simulink model "Demo_TA_cs"  (R2014b)
settings: Solver=FixedStepDiscrete  StartTime=0.0  StopTime=5  FixedStep=1/60  RelTol=1e-3
PreLoadFcn:
  | mbxruntime.callbacks.PreLoadFcn(bdroot);
  | check_NUTS_defined
  | 
  | assignin('base',['model_closed_' bdroot],false);
PostLoadFcn:
  | mbxruntime.callbacks.PostLoadFcn(bdroot);
InitFcn:
  | mbxruntime.callbacks.InitFcn(bdroot);
StartFcn:
  | mbxruntime.callbacks.StartFcn(bdroot);
  | 
  | open_system([bdroot '/Mazda_RX8_1/Scope']);
StopFcn:
  | mbxruntime.callbacks.StopFcn(bdroot);;
  | 
model workspace: external: MAT-File .\Demo_TA_cs_hws.mat (data not in the file)
undefined symbols (not defined in the file or in its folder): DriftAzimuthGaussianSigma, DriftAzimuthGaussianSigmaDefined, NoiseAzimuthIllumination, NoiseAzimuthIlluminationDefined, NoiseAzimuthReflection, NoiseAzimuthReflectionDefined, NoiseRange, NoiseRangeDefined, NoiseRangeType, NoiseRangeTypeDefined
undefined symbols (not defined in the file): Demo_TA_cs_Box_1_Dynamics_Empty_STATE_Box_1_Pitch0, Demo_TA_cs_Box_1_Dynamics_Empty_STATE_Box_1_Roll0, Demo_TA_cs_Box_1_Dynamics_Empty_STATE_Box_1_x0, Demo_TA_cs_Box_1_Dynamics_Empty_STATE_Box_1_y0, Demo_TA_cs_Box_1_Dynamics_Empty_STATE_Box_1_Yaw0, Demo_TA_cs_Box_1_Dynamics_Empty_STATE_Box_1_z0, Demo_TA_cs_Box_2_Dynamics_Empty_STATE_Box_2_Pitch0, Demo_TA_cs_Box_2_Dynamics_Empty_STATE_Box_2_Roll0, Demo_TA_cs_Box_2_Dynamics_Empty_STATE_Box_2_x0, Demo_TA_cs_Box_2_Dynamics_Empty_STATE_Box_2_y0, Demo_TA_cs_Box_2_Dynamics_Empty_STATE_Box_2_Yaw0, Demo_TA_cs_Box_2_Dynamics_Empty_STATE_Box_2_z0, Demo_TA_cs_Box_3_Dynamics_Empty_STATE_Box_3_Pitch0, Demo_TA_cs_Box_3_Dynamics_Empty_STATE_Box_3_Roll0, Demo_TA_cs_Box_3_Dynamics_Empty_STATE_Box_3_x0, Demo_TA_cs_Box_3_Dynamics_Empty_STATE_Box_3_y0, Demo_TA_cs_Box_3_Dynamics_Empty_STATE_Box_3_Yaw0, Demo_TA_cs_Box_3_Dynamics_Empty_STATE_Box_3_z0, Demo_TA_cs_Mazda_RX8_1_Dynamics_Empty_STATE_Mazda_RX8_1_Pitch0, Demo_TA_cs_Mazda_RX8_1_Dynamics_Empty_STATE_Mazda_RX8_1_Roll0, Demo_TA_cs_Mazda_RX8_1_Dynamics_Empty_STATE_Mazda_RX8_1_x0, Demo_TA_cs_Mazda_RX8_1_Dynamics_Empty_STATE_Mazda_RX8_1_y0, Demo_TA_cs_Mazda_RX8_1_Dynamics_Empty_STATE_Mazda_RX8_1_Yaw0, Demo_TA_cs_Mazda_RX8_1_Dynamics_Empty_STATE_Mazda_RX8_1_z0
libraries: PreScanSimulinkLibrary x8, PreScanUsefulBlocks x1
(part 1 of 2)
CloseFcn:
  | mbxruntime.callbacks.CloseFcn(bdroot);
  | evalin('base',['clear model_closed_' bdroot]);
settings Model: Creator=PRESCAN  LastModifiedBy=jenkins
settings DataIOCC: SignalLoggingSaveFormat=ModelDataLogs
settings OptimizationCC: InlineParams=on  ExpressionDepthLimit=2147483647  InitFltsAndDblsToZero=on
settings DebuggingCC: SaveWithParameterizedLinksMsg=none  UnderspecifiedInitializationDetection=Classic  MergeDetectMultiDrivingBlocksExec=none  SignalResolutionControl=TryResolveAllWithWarning  SolverPrmCheckMsg=none  MultiTaskDSMMsg=warning  MultiTaskCondExecSysMsg=none  FcnCallInpInsideContextMsg=UseLocalSettings  StateNameClashWarn=warning
settings ModelReferenceCC: UpdateModelReferenceTargets=IfOutOfDate
settings SFSimCC: SimParseCustomCode=off
settings SFSimCC: SimCustomHeaderCode=|
  | #include "prescan.h"
  | #include "prescan_platform.h"
settings RTWCC: IncludeERTFirstTime=on
settings GRTTargetCC: TargetFcnLib=ansi_tfl_tmw.mat  CombineOutputUpdateFcns=off  GRTInterface=on

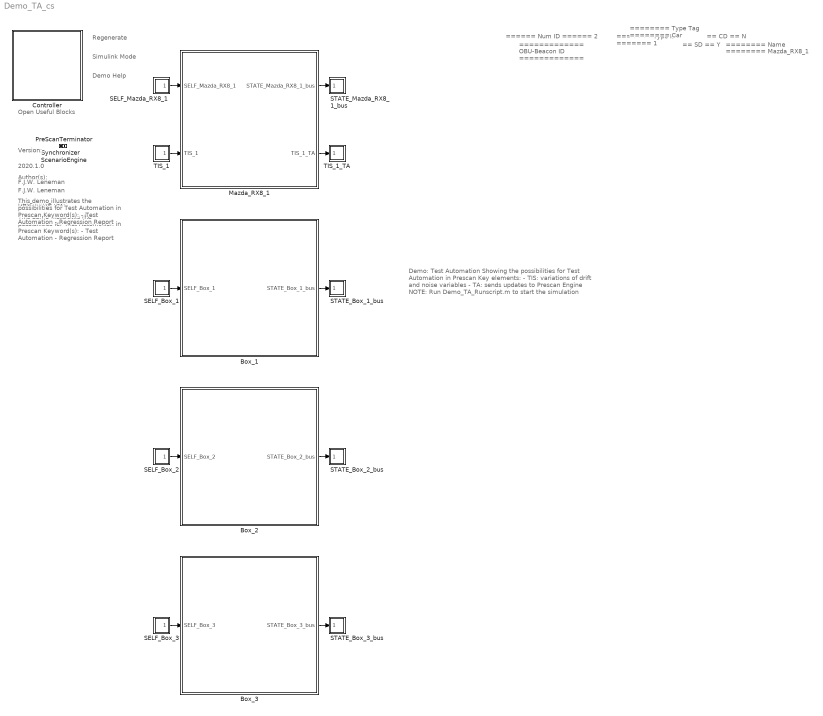
== system Demo_TA_cs ==
  note: Regenerate
  note: Simulink Mode
  note: Open Useful Blocks
  note: 2020.1.0
  note: Version:
  note: Author(s):
  note: F.J.W. Leneman
  note: Descriptive text:
  note: This demo illustrates the
      | possibilities for Test Automation
      | in Prescan
      |
      |
      |
      | Keyword(s):
      |
      | - Test Automation
      |
      | - Regression Report
  note: Demo Help
  note: Demo: Test Automation
      | Showing the possibilities for Test Automation in Prescan
      |
      | Key elements:
      | - TIS: variations of drift and noise variables
      | - TA: sends updates to Prescan Engine
      |
      | NOTE:
      | Run Demo_TA_Runscript.m to start the simulation
  note: This demo illustrates the
      | possibilities for Test Automation
      | in Prescan
      |
      |
      |
      | Keyword(s):
      |
      | - Test Automation
      |
      | - Regression Report
  note: F.J.W. Leneman
  note: ======
      | Num ID
      | ======
      | 2
  note: =============
      | OBU-Beacon ID
      | =============
  note: =======
      | Type ID
      | =======
      | 1
  note: ========
      | Type Tag
      | ========
      | Car
  note: ==
      | SD
      | ==
      | Y
  note: ==
      | CD
      | ==
      | N
  note: ========
      | Name
      | ========
      | Mazda_RX8_1
  Box_1 : Subsystem  Tag=WorldObjectSubSystem  InitFcn=UniqueId = '8';
      mask init:
      | imagePath=which('Box.jpg');
      mask Display: image(imread(imagePath));color('white');text(0, 0, ' ID=3\n')
  Box_2 : Subsystem  Tag=WorldObjectSubSystem  InitFcn=UniqueId = '9';
      mask init:
      | imagePath=which('Box.jpg');
      mask Display: image(imread(imagePath));color('white');text(0, 0, ' ID=4\n')
  Box_3 : Subsystem  Tag=WorldObjectSubSystem  InitFcn=UniqueId = '10';
      mask init:
      | imagePath=which('Box.jpg');
      mask Display: image(imread(imagePath));color('white');text(0, 0, ' ID=5\n')
  Controller : Subsystem  Description=8A3CD2955739A82C886C20AE3E253D78460D53180EE2C1B14CC08DF75A70BE77  Priority=-1  LoadFcn=load PreScanControllerData  mask(PreScan Simulation Controller){prescanversion='2020.1.0', ModelReferencing=off, TimeStep=1/60, ControlMode=0, PreScanExecutionMode=on, ControllerCount=0, ControllerIndex=0, ControllerOptions=''}
      mask prompts: prescanversion "PreScan Version"; ModelReferencing "Use Model Referencing"; TimeStep "Upload Period [s]"; ControlMode "Control Mode"; PreScanExecutionMode "Execution Mode"; ControllerCount "Controller Count"; ControllerIndex "Controller Index"; ControllerOptions "Controller Options"
      mask help:
      | Please do not remove this block from the compilation sheet,
      | as it connects the model to the PreScan environment.
      mask init:
      | model = bdroot(gcb);
      | ExperimentFile = mbxruntime.findExperimentFile(model,true); %relative path
      | 
      | [d1, d2, d3, prescandata] = prescan_Settings();
      | ModelDepo = fullfile(prescandata,'ModelDepo'); 
      | 
      | RTmode = mbxruntime.getRTMode(model);
      | 
      | SimulationMode = get_param(bdroot,'SimulationMode');
      | if strcmp(SimulationMode, 'rapid-accelerator')
      |     SimulationMode = 'external';
      | end
      | TargetName = get_param(bdroot,'SystemTargetFile');
      settings: ModelCloseFcn=assignin('base',['model_closed_' bdroot],true);
      mask Help: eval('openHelp(812)')
      mask Display: image(imread('prescanlogo.ico'))
  Mazda_RX8_1 : Subsystem  Tag=WorldObjectSubSystem  InitFcn=UniqueId = '6';
      mask init:
      | modelPath = GenericModelHelper.getGenericModelFilePath('ModelDepo','Vehicles\Mazda_RX8\Mazda_RX8.pgmb','1e55a2e40efa576b7f4fb93bae35d605');imagePath = GenericModelHelper.getCompilationPicture(modelPath, 'Mazda_RX8_HighPoly.png');
      mask Display: image(imread(imagePath));color('white');text(0, 0, ' ID=2\n')
  PreScanTerminator : Subsystem  Tag=PreScanTerminator  Priority=999  LoadFcn=load PrescanTerminatorData  mask(PreScan Simulation Terminator){TimeStep=1/60}
      mask prompts: TimeStep "Upload Period [s]"
      mask help:
      | Please do not remove this block from the compilation sheet as it
      | connects the model to the PreScan environment.
      mask Help: eval('openHelp(812)')
      mask Display: image(imread('prescanlogo.ico'))
  SELF_Box_1 : Subsystem  Tag=sensor/SelfPort  Priority=30  LoadFcn=load('PreScanSelfSensorData.mat')  mask(PreScan Source Block: SELF){}
      mask help:
      | The SELF port shows (state) information of the actor itself. The outputs are position in the experiment's axis system and the GPS coordinates, and the object's absolute velocity and compass heading.
      |
      | For more information, please click Help.
      settings: OpenFcn=open_system([gcb '/Sensor'],'mask')
      mask Help: eval('openHelp(462)')
      mask Display: image(imread('GPS.png'))
  SELF_Box_2 : Subsystem  Tag=sensor/SelfPort  Priority=30  LoadFcn=load('PreScanSelfSensorData.mat')  mask(PreScan Source Block: SELF){}
      mask help:
      | The SELF port shows (state) information of the actor itself. The outputs are position in the experiment's axis system and the GPS coordinates, and the object's absolute velocity and compass heading.
      |
      | For more information, please click Help.
      settings: OpenFcn=open_system([gcb '/Sensor'],'mask')
      mask Help: eval('openHelp(462)')
      mask Display: image(imread('GPS.png'))
  SELF_Box_3 : Subsystem  Tag=sensor/SelfPort  Priority=30  LoadFcn=load('PreScanSelfSensorData.mat')  mask(PreScan Source Block: SELF){}
      mask help:
      | The SELF port shows (state) information of the actor itself. The outputs are position in the experiment's axis system and the GPS coordinates, and the object's absolute velocity and compass heading.
      |
      | For more information, please click Help.
      settings: OpenFcn=open_system([gcb '/Sensor'],'mask')
      mask Help: eval('openHelp(462)')
      mask Display: image(imread('GPS.png'))
  SELF_Mazda_RX8_1 : Subsystem  Tag=sensor/SelfPort  Priority=30  LoadFcn=load('PreScanSelfSensorData.mat')  mask(PreScan Source Block: SELF){}
      mask help:
      | The SELF port shows (state) information of the actor itself. The outputs are position in the experiment's axis system and the GPS coordinates, and the object's absolute velocity and compass heading.
      |
      | For more information, please click Help.
      settings: OpenFcn=open_system([gcb '/Sensor'],'mask')
      mask Help: eval('openHelp(462)')
      mask Display: image(imread('GPS.png'))
  STATE_Box_1_bus : Subsystem  Tag=actuator/StatePort  Priority=0  LoadFcn=load('PreScanStateActuatorData.mat')  mask(PreScan Sink Block: State){}
      mask help:
      | The Actor State contains a vector signal of size (9x1), containing the following signals:
      |
      | -  Position    	(x,y,z)             	[m]
      | -  Velocity    	(vx,vy,vz)         	[m/s]
      | -  Angles       	(Roll, Pitch, Yaw)	[rad]
      |
      | The Actor state is defined in the global axis system.
      | The state is superponed on the Initial position defined in the GUI.
      |
      | For more information, please click Help.
      settings: OpenFcn=open_system([gcb '/Actuator'],'mask')
      mask Help: eval('openHelp(222)')
      mask Display: image(imread('State.png'))
  STATE_Box_2_bus : Subsystem  Tag=actuator/StatePort  Priority=0  LoadFcn=load('PreScanStateActuatorData.mat')  mask(PreScan Sink Block: State){}
      mask help:
      | The Actor State contains a vector signal of size (9x1), containing the following signals:
      |
      | -  Position    	(x,y,z)             	[m]
      | -  Velocity    	(vx,vy,vz)         	[m/s]
      | -  Angles       	(Roll, Pitch, Yaw)	[rad]
      |
      | The Actor state is defined in the global axis system.
      | The state is superponed on the Initial position defined in the GUI.
      |
      | For more information, please click Help.
      settings: OpenFcn=open_system([gcb '/Actuator'],'mask')
      mask Help: eval('openHelp(222)')
      mask Display: image(imread('State.png'))
  STATE_Box_3_bus : Subsystem  Tag=actuator/StatePort  Priority=0  LoadFcn=load('PreScanStateActuatorData.mat')  mask(PreScan Sink Block: State){}
      mask help:
      | The Actor State contains a vector signal of size (9x1), containing the following signals:
      |
      | -  Position    	(x,y,z)             	[m]
      | -  Velocity    	(vx,vy,vz)         	[m/s]
      | -  Angles       	(Roll, Pitch, Yaw)	[rad]
      |
      | The Actor state is defined in the global axis system.
      | The state is superponed on the Initial position defined in the GUI.
      |
      | For more information, please click Help.
      settings: OpenFcn=open_system([gcb '/Actuator'],'mask')
      mask Help: eval('openHelp(222)')
      mask Display: image(imread('State.png'))
  STATE_Mazda_RX8_1_bus : Subsystem  Tag=actuator/StatePort  Priority=0  LoadFcn=load('PreScanStateActuatorData.mat')  mask(PreScan Sink Block: State){}
      mask help:
      | The Actor State contains a vector signal of size (9x1), containing the following signals:
      |
      | -  Position    	(x,y,z)             	[m]
      | -  Velocity    	(vx,vy,vz)         	[m/s]
      | -  Angles       	(Roll, Pitch, Yaw)	[rad]
      |
      | The Actor state is defined in the global axis system.
      | The state is superponed on the Initial position defined in the GUI.
      |
      | For more information, please click Help.
      settings: OpenFcn=open_system([gcb '/Actuator'],'mask')
      mask Help: eval('openHelp(222)')
      mask Display: image(imread('State.png'))
  ScenarioEngine : Subsystem  Tag=PreScanOpenScenarioBlock  Priority=10  LoadFcn=load PrescanSynchronizeData  mask(PreScan Simulation Core Block){TimeStep=1/60}
      mask prompts: TimeStep "Timestep [s]"
      mask help:
      | Please do not remove this block from the PreScan compilation sheet,
      | as it contains essential configuration parameters for a PreScan simulation.
      settings: DeleteFcn=PreScanBlockDeleteFcn;
      mask Display: image(imread('prescanlogo.ico'))
  Synchronizer : Subsystem  Tag=PreScanSynchronizer  Priority=20  LoadFcn=load PrescanSynchronizeData  mask(PreScan Simulation Core Block){TimeStep=1/60}
      mask prompts: TimeStep "Timestep [s]"
      mask help:
      | Please do not remove this block from the PreScan compilation sheet,
      | as it contains essential configuration parameters for a PreScan simulation.
      settings: DeleteFcn=PreScanBlockDeleteFcn;
      mask Display: image(imread('prescanlogo.ico'))
  TIS_1 : Subsystem  Tag=sensor/TIS  Priority=30  LoadFcn=load('PrescanScannerSensorData.mat');load('PrescanScannerSensorMessage.mat')  mask(PreScan Source Block: Technology Independent Sensor (TIS)){}
      mask help:
      | The Technology Independent Sensor (TIS) provides a sensor with all sensor-related influence factors (like noise, drift and accuracy) without being technology specific (like radar and lidar). The TIS detects the closest point on the geometry of an object.
      |
      | For more information, please click Help.
      settings: OpenFcn=open_system([gcb '/Sensor'],'mask')
      mask Help: eval('openHelp(449)')
      mask Display: image(imread('TIS.png'))
  TIS_1_TA : Subsystem  Tag=actuator/TIS_TA  Priority=0  LoadFcn=load('PrescanScannerSensorTA.mat')  mask(TIS Test Automation){}
      mask help:
      | The TA Sink block updates the Test Automation variables in the Simulation.
      |
      | Note: All angles are expressed in degrees
      |
      | Remarks:
      | TIS: Drift Type:
      |   0: None
      |   1: Gaussian
      |   2: Unidirectional
      |
      | TIS: Noise Type:
      |   0: Additive
      |   1: Multiplicative
      |
      | AIR: Detection Type:
      |   0: BoundingBox
      |   1: Bounding Box Center
      |   2: CenterOfGravity
      |
      | Antenna Tx: Range
      |   -1: Infinite
      |
      | For more information, please click Help.
      settings: OpenFcn=open_system([gcb '/Actuator'],'mask')
      mask Help: eval('openHelp(633)')
      mask Display: image(imread('TA.png'))
  wires:
  Mazda_RX8_1/1(STATE_Mazda_RX8_1_bus) -> STATE_Mazda_RX8_1_bus/1(STATE_Mazda_RX8_1_bus)
  SELF_Mazda_RX8_1/1(SELF_Mazda_RX8_1) -> Mazda_RX8_1/1(SELF_Mazda_RX8_1)
  TIS_1/1(TIS_1) -> Mazda_RX8_1/2(TIS_1)
  Mazda_RX8_1/2(TIS_1_TA) -> TIS_1_TA/1(TIS_1_TA)
  Box_1/1(STATE_Box_1_bus) -> STATE_Box_1_bus/1(STATE_Box_1_bus)
  SELF_Box_1/1(SELF_Box_1) -> Box_1/1(SELF_Box_1)
  Box_2/1(STATE_Box_2_bus) -> STATE_Box_2_bus/1(STATE_Box_2_bus)
  SELF_Box_2/1(SELF_Box_2) -> Box_2/1(SELF_Box_2)
  Box_3/1(STATE_Box_3_bus) -> STATE_Box_3_bus/1(STATE_Box_3_bus)
  SELF_Box_3/1(SELF_Box_3) -> Box_3/1(SELF_Box_3)

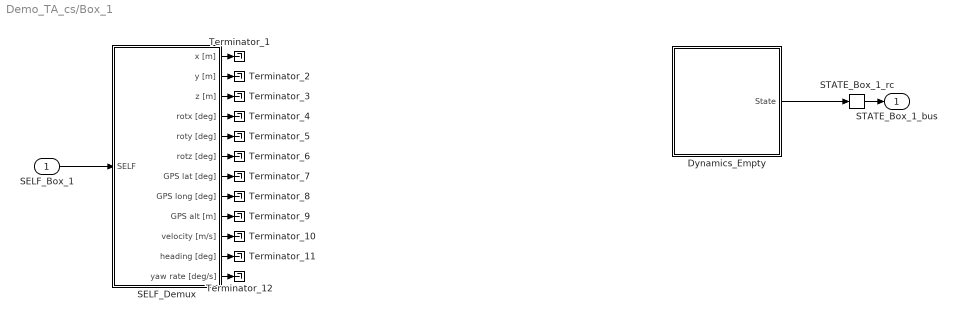
== system Demo_TA_cs/Box_1 ==
  SELF_Box_1 : Inport  Tag=inport/SelfPort  OutDataTypeStr=Bus: PRESCAN_SELFSENSORDATA  PortDimensions=1  SampleTime=1/60  BusOutputAsStruct=on
  Dynamics_Empty : Subsystem  Tag=Dynamics_Empty
      mask Help: eval('openHelp(202)')
      mask Display: port_label('output', 1, 'State');text(0,0,' Empty\n')
  SELF_Demux : Subsystem  Tag=demux/SelfPort  mask(PreScan Demux Block:){}
      mask help:
      | The SELF port shows (state) information of the actor itself. The outputs are position in the experiment's axis system and the GPS coordinates, and the object's absolute velocity and compass heading.
      |
      | For more information, please click Help.
      settings: DeleteFcn=PreScanBlockDeleteFcn;
      mask Help: eval('openHelp(462)')
      mask Display:
      | port_label('output',1,'x [m]')
      | port_label('output',2,'y [m]')
      | port_label('output',3,'z [m]','texmode','on')
      | port_label('output',4,'Rotx [deg]','texmode','on')
      | port_label('output',5,'Roty [deg]','texmode','on')
      | port_label('output',6,'Rotz [deg]','texmode','on')
      | port_label('output',7,'GPS lat [deg]','texmode','on')
      | port_label('output',8,'GPS long [deg]','texmode','on')
      | port_label('output',9,'GPS alt [m]','texmode','on')
      | port_label('output',10,'Velocity [m/s]')
      | port_label('output',11,'Heading [deg]')
      | port_label('output',12,'Yaw rate [deg/s]')
  STATE_Box_1_rc : RateTransition  Tag=mux_rc/StatePort  OutPortSampleTimeOpt=Inherit
  Terminator_{1..12} (12 alike) : Terminator
  STATE_Box_1_bus : Outport  Tag=outport/StatePort  OutDataTypeStr=Bus: PRESCAN_STATEACTUATORDATA  PortDimensions=1  SampleTime=1/60
  wires:
  STATE_Box_1_rc/1 -> STATE_Box_1_bus/1
  SELF_Box_1/1 -> SELF_Demux/1(SELF)
  Dynamics_Empty/1(State) -> STATE_Box_1_rc/1
  SELF_Demux/1(x [m]) -> Terminator_1/1
  SELF_Demux/2(y [m]) -> Terminator_2/1
  SELF_Demux/3(z [m]) -> Terminator_3/1
  SELF_Demux/4(rotx [deg]) -> Terminator_4/1
  SELF_Demux/5(roty [deg]) -> Terminator_5/1
  SELF_Demux/6(rotz [deg]) -> Terminator_6/1
  SELF_Demux/7(GPS lat [deg]) -> Terminator_7/1
  SELF_Demux/8(GPS long [deg]) -> Terminator_8/1
  SELF_Demux/9(GPS alt [m]) -> Terminator_9/1
  SELF_Demux/10(velocity [m/s]) -> Terminator_10/1
  SELF_Demux/11(heading [deg]) -> Terminator_11/1
  SELF_Demux/12(yaw rate [deg/s]) -> Terminator_12/1

== system Demo_TA_cs/Box_2 ==
  SELF_Box_2 : Inport  Tag=inport/SelfPort  OutDataTypeStr=Bus: PRESCAN_SELFSENSORDATA  PortDimensions=1  SampleTime=1/60  BusOutputAsStruct=on
  Dynamics_Empty : Subsystem  Tag=Dynamics_Empty
      mask Help: eval('openHelp(202)')
      mask Display: port_label('output', 1, 'State');text(0,0,' Empty\n')
  SELF_Demux : Subsystem  Tag=demux/SelfPort  mask(PreScan Demux Block:){}
      mask help:
      | The SELF port shows (state) information of the actor itself. The outputs are position in the experiment's axis system and the GPS coordinates, and the object's absolute velocity and compass heading.
      |
      | For more information, please click Help.
      settings: DeleteFcn=PreScanBlockDeleteFcn;
      mask Help: eval('openHelp(462)')
      mask Display:
      | port_label('output',1,'x [m]')
      | port_label('output',2,'y [m]')
      | port_label('output',3,'z [m]','texmode','on')
      | port_label('output',4,'Rotx [deg]','texmode','on')
      | port_label('output',5,'Roty [deg]','texmode','on')
      | port_label('output',6,'Rotz [deg]','texmode','on')
      | port_label('output',7,'GPS lat [deg]','texmode','on')
      | port_label('output',8,'GPS long [deg]','texmode','on')
      | port_label('output',9,'GPS alt [m]','texmode','on')
      | port_label('output',10,'Velocity [m/s]')
      | port_label('output',11,'Heading [deg]')
      | port_label('output',12,'Yaw rate [deg/s]')
  STATE_Box_2_rc : RateTransition  Tag=mux_rc/StatePort  OutPortSampleTimeOpt=Inherit
  Terminator_{1..12} (12 alike) : Terminator
  STATE_Box_2_bus : Outport  Tag=outport/StatePort  OutDataTypeStr=Bus: PRESCAN_STATEACTUATORDATA  PortDimensions=1  SampleTime=1/60
  wires:
  STATE_Box_2_rc/1 -> STATE_Box_2_bus/1
  SELF_Box_2/1 -> SELF_Demux/1(SELF)
  Dynamics_Empty/1(State) -> STATE_Box_2_rc/1
  SELF_Demux/1(x [m]) -> Terminator_1/1
  SELF_Demux/2(y [m]) -> Terminator_2/1
  SELF_Demux/3(z [m]) -> Terminator_3/1
  SELF_Demux/4(rotx [deg]) -> Terminator_4/1
  SELF_Demux/5(roty [deg]) -> Terminator_5/1
  SELF_Demux/6(rotz [deg]) -> Terminator_6/1
  SELF_Demux/7(GPS lat [deg]) -> Terminator_7/1
  SELF_Demux/8(GPS long [deg]) -> Terminator_8/1
  SELF_Demux/9(GPS alt [m]) -> Terminator_9/1
  SELF_Demux/10(velocity [m/s]) -> Terminator_10/1
  SELF_Demux/11(heading [deg]) -> Terminator_11/1
  SELF_Demux/12(yaw rate [deg/s]) -> Terminator_12/1

== system Demo_TA_cs/Box_3 ==
  SELF_Box_3 : Inport  Tag=inport/SelfPort  OutDataTypeStr=Bus: PRESCAN_SELFSENSORDATA  PortDimensions=1  SampleTime=1/60  BusOutputAsStruct=on
  Dynamics_Empty : Subsystem  Tag=Dynamics_Empty
      mask Help: eval('openHelp(202)')
      mask Display: port_label('output', 1, 'State');text(0,0,' Empty\n')
  SELF_Demux : Subsystem  Tag=demux/SelfPort  mask(PreScan Demux Block:){}
      mask help:
      | The SELF port shows (state) information of the actor itself. The outputs are position in the experiment's axis system and the GPS coordinates, and the object's absolute velocity and compass heading.
      |
      | For more information, please click Help.
      settings: DeleteFcn=PreScanBlockDeleteFcn;
      mask Help: eval('openHelp(462)')
      mask Display:
      | port_label('output',1,'x [m]')
      | port_label('output',2,'y [m]')
      | port_label('output',3,'z [m]','texmode','on')
      | port_label('output',4,'Rotx [deg]','texmode','on')
      | port_label('output',5,'Roty [deg]','texmode','on')
      | port_label('output',6,'Rotz [deg]','texmode','on')
      | port_label('output',7,'GPS lat [deg]','texmode','on')
      | port_label('output',8,'GPS long [deg]','texmode','on')
      | port_label('output',9,'GPS alt [m]','texmode','on')
      | port_label('output',10,'Velocity [m/s]')
      | port_label('output',11,'Heading [deg]')
      | port_label('output',12,'Yaw rate [deg/s]')
  STATE_Box_3_rc : RateTransition  Tag=mux_rc/StatePort  OutPortSampleTimeOpt=Inherit
  Terminator_{1..12} (12 alike) : Terminator
  STATE_Box_3_bus : Outport  Tag=outport/StatePort  OutDataTypeStr=Bus: PRESCAN_STATEACTUATORDATA  PortDimensions=1  SampleTime=1/60
  wires:
  STATE_Box_3_rc/1 -> STATE_Box_3_bus/1
  SELF_Box_3/1 -> SELF_Demux/1(SELF)
  Dynamics_Empty/1(State) -> STATE_Box_3_rc/1
  SELF_Demux/1(x [m]) -> Terminator_1/1
  SELF_Demux/2(y [m]) -> Terminator_2/1
  SELF_Demux/3(z [m]) -> Terminator_3/1
  SELF_Demux/4(rotx [deg]) -> Terminator_4/1
  SELF_Demux/5(roty [deg]) -> Terminator_5/1
  SELF_Demux/6(rotz [deg]) -> Terminator_6/1
  SELF_Demux/7(GPS lat [deg]) -> Terminator_7/1
  SELF_Demux/8(GPS long [deg]) -> Terminator_8/1
  SELF_Demux/9(GPS alt [m]) -> Terminator_9/1
  SELF_Demux/10(velocity [m/s]) -> Terminator_10/1
  SELF_Demux/11(heading [deg]) -> Terminator_11/1
  SELF_Demux/12(yaw rate [deg/s]) -> Terminator_12/1

== system Demo_TA_cs/Controller ==
  Terminator : Terminator
  sfun_Controller : S-Function  FunctionName=sfun_Controller  Parameters=SParameter1, SParameter2, SParameter3, SParameter4, SParameter5, SParameter6, SParameter7, SParameter8, SParameter9, SParameter10, SampleTime  EnableBusSupport=off  mask(Legacy Function){SFunctionSpec=void prescan_outputFcn(void** work1, PRESCAN_CONTROLLERDATA y1[1]), SParameter1=uint8([ExperimentFile 0]), SParameter2=uint8([ModelDepo 0]), SParameter3=uint8([ControllerOptions 0]), SParameter4=RTmode, SParameter5=PreScanExecutionMode, SParameter6=ControlMode, SParameter7=ControllerCount, SParameter8=ControllerIndex, SParameter9=uint8([SimulationMode 0]), SParameter10=uint8([TargetName 0]), SampleTime=TimeStep, ShowSpec=on}
      mask prompts: SParameter1 "P1:"; SParameter2 "P2:"; SParameter3 "P3:"; SParameter4 "P4:"; SParameter5 "P5:"; SParameter6 "P6:"; SParameter7 "P7:"; SParameter8 "P8:"; SParameter9 "P9:"; SParameter10 "P10:"; SampleTime "Sample time (-1 for inherited):"; ShowSpec "Display function specification"
      mask help:
      | This block allows you to call the legacy functions specified by the following Legacy Code Tool definition:
      | def.SFunctionName = 'sfun_Controller';
      | def.OutputFcnSpec = 'void prescan_outputFcn(void** work1, PRESCAN_CONTROLLERDATA y1[1])';
      | def.StartFcnSpec = 'void prescan_startFcn(void ** work1, uint8 p1[], uint8 p2[], uint8 p3[], double p4, double p5, double p6, double p7, double p8, uint8 p9[], uint8 p10[])';
      | def.TerminateFcnSpec = 'void prescan_terminateFcn(void** work1)';
      | def.HeaderFiles = {'prescan_controller_data.h', 'prescan_SFunLibrary.h', 'prescan_CreateLogHandler.h', 'prescan_CreateErrorHandler.h', 'prescan_modify.h', 'ModuleDLL.h'};
      | def.SourceFiles = {'prescan_MexLogHandler.c', 'prescan_SimStructErrorHandler.c', 'prescan_LogHandler.c', 'prescan_ErrorHandler.c', 'prescan_Modify.c'};
      | def.HostLibFiles = {'sensorinterfaced.lib'};
      | def.TargetLibFiles = {'sensorinterfaced.so'};
      | def.IncPaths = {'.', 'C:\projects\prescan\rt_vislibrary\vis\..\pimp\include\sensors\InterfaceRTW'};
      | def.SrcPaths = {'C:\projects\prescan\rt_vislibrary\vis\..\pimp\include\sensors\InterfaceRTW', 'C:\projects\prescan\rt_vislibrary\vis\..\pimp\include\sensors\InterfaceRTW\ccurrt'};
      | def.LibPaths = {'C:\\projects\\prescan\\vislibrary_build\lib'};
      | def.SampleTime = 'parameterized';
      mask Help: <p>This block was generated automatically by the Legacy Code Tool. For detailed help on this tool, call<a href="matlab:legacy_code('help')"> legacy_code('help')</a>.</p>
      mask Callback ShowSpec:
      | if strcmp(get_param(gcbh, 'ShowSpec'), 'on')
      |   set_param(gcbh, 'MaskDisplay', sprintf('fprintf(''%s'');', get_param(gcbh, 'SFunctionSpec')));
      | else
      |   set_param(gcbh, 'MaskDisplay', sprintf('fprintf(''%s'');', get_param(gcbh, 'FunctionName')));
      | end
      mask Display: fprintf('void prescan_outputFcn(void** work1, PRESCAN_CONTROLLERDATA y1[1])');
  wires:
  sfun_Controller/1 -> Terminator/1

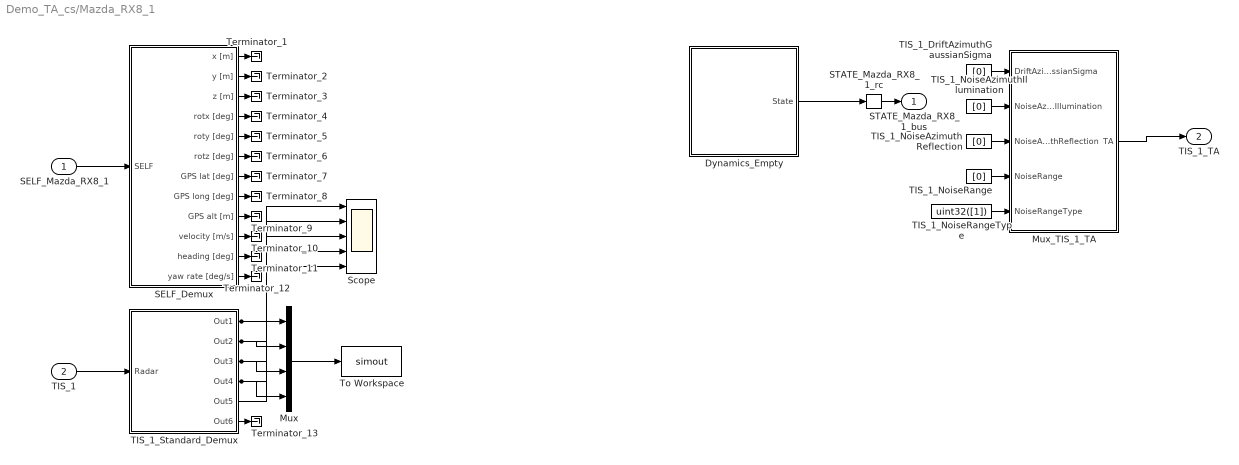
== system Demo_TA_cs/Mazda_RX8_1 ==
  SELF_Mazda_RX8_1 : Inport  Tag=inport/SelfPort  OutDataTypeStr=Bus: PRESCAN_SELFSENSORDATA  PortDimensions=1  SampleTime=1/60  BusOutputAsStruct=on
  TIS_1 : Inport  Tag=inport/TIS  Port=2  OutDataTypeStr=Bus: PRESCAN_SCANNERSENSOR_MESSAGE  PortDimensions=1  SampleTime=1/60  BusOutputAsStruct=on
  Dynamics_Empty : Subsystem  Tag=Dynamics_Empty
      mask Help: eval('openHelp(202)')
      mask Display: port_label('output', 1, 'State');text(0,0,' Empty\n')
  Mux : Mux
  Mux_TIS_1_TA : Subsystem  Tag=mux/TIS_TA
  SELF_Demux : Subsystem  Tag=demux/SelfPort  mask(PreScan Demux Block:){}
      mask help:
      | The SELF port shows (state) information of the actor itself. The outputs are position in the experiment's axis system and the GPS coordinates, and the object's absolute velocity and compass heading.
      |
      | For more information, please click Help.
      settings: DeleteFcn=PreScanBlockDeleteFcn;
      mask Help: eval('openHelp(462)')
      mask Display:
      | port_label('output',1,'x [m]')
      | port_label('output',2,'y [m]')
      | port_label('output',3,'z [m]','texmode','on')
      | port_label('output',4,'Rotx [deg]','texmode','on')
      | port_label('output',5,'Roty [deg]','texmode','on')
      | port_label('output',6,'Rotz [deg]','texmode','on')
      | port_label('output',7,'GPS lat [deg]','texmode','on')
      | port_label('output',8,'GPS long [deg]','texmode','on')
      | port_label('output',9,'GPS alt [m]','texmode','on')
      | port_label('output',10,'Velocity [m/s]')
      | port_label('output',11,'Heading [deg]')
      | port_label('output',12,'Yaw rate [deg/s]')
  STATE_Mazda_RX8_1_rc : RateTransition  Tag=mux_rc/StatePort  OutPortSampleTimeOpt=Inherit
  Scope : Scope  NumInputPorts=5
      settings: YMin=-5~-5~-5~-5~-5  YMax=5~5~5~5~5  SaveName=ScopeData2
  TIS_1_DriftAzimuthGaussianSigma : Constant  Tag=TIS_1_DriftAzimuthGaussianSigma  Value=[0]
  TIS_1_NoiseAzimuthIllumination : Constant  Tag=TIS_1_NoiseAzimuthIllumination  Value=[0]
  TIS_1_NoiseAzimuthReflection : Constant  Tag=TIS_1_NoiseAzimuthReflection  Value=[0]
  TIS_1_NoiseRange : Constant  Tag=TIS_1_NoiseRange  Value=[0]
  TIS_1_NoiseRangeType : Constant  Tag=TIS_1_NoiseRangeType  Value=uint32([1])
  TIS_1_Standard_Demux : Subsystem  Tag=demux/TIS/Standard  TreatAsAtomicUnit=on  mask(PreScan Demux Block: TIS){MAXMESSAGES=1}
      mask prompts: MAXMESSAGES "Number of Objects"
      mask Help: eval('openHelp(449)')
      mask Display:
      | port_label('input',1,'TIS')
      | port_label('output',1,'Beam ID [-]')
      | port_label('output',2,'Range [m]')
      | port_label('output',3,'{\theta} [deg]','texmode','on')
      | port_label('output',4,'{\phi} [deg]','texmode','on')
      | port_label('output',5,'Target ID [-]','texmode','on')
      | port_label('output',6,'TIS Data','texmode','on')
  Terminator_{1..13} (13 alike) : Terminator
  To Workspace : ToWorkspace  VariableName=simout  SampleTime=-1
  STATE_Mazda_RX8_1_bus : Outport  Tag=outport/StatePort  OutDataTypeStr=Bus: PRESCAN_STATEACTUATORDATA  PortDimensions=1  SampleTime=1/60
  TIS_1_TA : Outport  Tag=outport/TIS_TA  Port=2  OutDataTypeStr=Bus: PRESCAN_SCANNERSENSOR_TA  PortDimensions=1  SampleTime=1/60
  wires:
  Mux/1 -> To Workspace/1
  TIS_1_Standard_Demux/1(Out1) -> Mux/1, Scope/1
  TIS_1_Standard_Demux/2(Out2) -> Mux/2, Scope/2
  TIS_1_Standard_Demux/3(Out3) -> Mux/3, Scope/3
  TIS_1_Standard_Demux/4(Out4) -> Mux/4, Scope/4
  TIS_1_Standard_Demux/5(Out5) -> Scope/5
  STATE_Mazda_RX8_1_rc/1 -> STATE_Mazda_RX8_1_bus/1
  SELF_Mazda_RX8_1/1 -> SELF_Demux/1(SELF)
  TIS_1/1 -> TIS_1_Standard_Demux/1(Radar)
  TIS_1_DriftAzimuthGaussianSigma/1 -> Mux_TIS_1_TA/1(DriftAzimuthGaussianSigma)
  TIS_1_NoiseAzimuthIllumination/1 -> Mux_TIS_1_TA/2(NoiseAzimuthIllumination)
  TIS_1_NoiseAzimuthReflection/1 -> Mux_TIS_1_TA/3(NoiseAzimuthReflection)
  TIS_1_NoiseRange/1 -> Mux_TIS_1_TA/4(NoiseRange)
  TIS_1_NoiseRangeType/1 -> Mux_TIS_1_TA/5(NoiseRangeType)
  Mux_TIS_1_TA/1(TA) -> TIS_1_TA/1
  Dynamics_Empty/1(State) -> STATE_Mazda_RX8_1_rc/1
  SELF_Demux/1(x [m]) -> Terminator_1/1
  SELF_Demux/2(y [m]) -> Terminator_2/1
  SELF_Demux/3(z [m]) -> Terminator_3/1
  SELF_Demux/4(rotx [deg]) -> Terminator_4/1
  SELF_Demux/5(roty [deg]) -> Terminator_5/1
  SELF_Demux/6(rotz [deg]) -> Terminator_6/1
  SELF_Demux/7(GPS lat [deg]) -> Terminator_7/1
  SELF_Demux/8(GPS long [deg]) -> Terminator_8/1
  SELF_Demux/9(GPS alt [m]) -> Terminator_9/1
  SELF_Demux/10(velocity [m/s]) -> Terminator_10/1
  SELF_Demux/11(heading [deg]) -> Terminator_11/1
  SELF_Demux/12(yaw rate [deg/s]) -> Terminator_12/1
  TIS_1_Standard_Demux/6(Out6) -> Terminator_13/1

== system Demo_TA_cs/PreScanTerminator ==
  Terminator : Terminator
  sfun_Terminator : S-Function  FunctionName=sfun_Terminator  Parameters=SampleTime  EnableBusSupport=off  mask(Legacy Function){SFunctionSpec=void prescan_terminator_outputFcn(void ** work1, PRESCAN_TERMINATORDATA y1[1]), SampleTime=TimeStep, ShowSpec=on}
      mask prompts: SampleTime "Sample time (-1 for inherited):"; ShowSpec "Display function specification"
      mask help:
      | This block allows you to call the legacy functions specified by the following Legacy Code Tool definition:
      | def.SFunctionName = 'sfun_Terminator';
      | def.OutputFcnSpec = 'void prescan_terminator_outputFcn(void ** work1, PRESCAN_TERMINATORDATA y1[1])';
      | def.StartFcnSpec = 'void prescan_terminator_startFcn(void ** work1)';
      | def.TerminateFcnSpec = 'void prescan_terminator_terminateFcn(void ** work1)';
      | def.HeaderFiles = {'prescan_terminator_data.h'};
      | def.HostLibFiles = {'sensorinterfaced.lib'};
      | def.IncPaths = {'src', 'C:\prescandev\vislibrary\vis\..\pimp\include\sensors\InterfaceRTW'};
      | def.SrcPaths = {'src'};
      | def.LibPaths = {'C:\\prescandev\\vislibrary_build\lib'};
      | def.SampleTime = 'parameterized';
      | def.Options.language = 'C';
      mask Help: <p>This block was generated automatically by the Legacy Code Tool. For detailed help on this tool, call<a href="matlab:legacy_code('help')"> legacy_code('help')</a>.</p>
      mask Callback ShowSpec:
      | if strcmp(get_param(gcbh, 'ShowSpec'), 'on')
      |   set_param(gcbh, 'MaskDisplay', sprintf('fprintf(''%s'');', get_param(gcbh, 'SFunctionSpec')));
      | else
      |   set_param(gcbh, 'MaskDisplay', sprintf('fprintf(''%s'');', get_param(gcbh, 'FunctionName')));
      | end
      mask Display: fprintf('void prescan_terminator_outputFcn(void ** work1, PRESCAN_TERMINATORDATA y1[1])');
  wires:
  sfun_Terminator/1 -> Terminator/1

== system Demo_TA_cs/SELF_Box_1 ==
  Sensor : S-Function  FunctionName=sfun_SelfSensor  Parameters=UniqueID, TimeStep  EnableBusSupport=off  mask(PreScan Source Block: SELF){UniqueID=8, TimeStep=1/60}
      mask prompts: UniqueID "Auto-Assigned: Unique ID"; TimeStep "Auto-Assigned: Upload Period [s]"
      mask help:
      | The SELF port shows (state) information of the actor itself. The outputs are position in the experiment's axis system and the GPS coordinates, and the object's absolute velocity and compass heading.
      |
      | For more information, please click Help.
      mask Help: eval('openHelp(462)')
      mask Display: image(imread('GPS.png'))
  SELF_Box_1 : Outport  Tag=outport/SelfPort  OutDataTypeStr=Bus: PRESCAN_SELFSENSORDATA  PortDimensions=1  SampleTime=1/60
  wires:
  Sensor/1 -> SELF_Box_1/1

== system Demo_TA_cs/SELF_Box_2 ==
  Sensor : S-Function  FunctionName=sfun_SelfSensor  Parameters=UniqueID, TimeStep  EnableBusSupport=off  mask(PreScan Source Block: SELF){UniqueID=9, TimeStep=1/60}
      mask prompts: UniqueID "Auto-Assigned: Unique ID"; TimeStep "Auto-Assigned: Upload Period [s]"
      mask help:
      | The SELF port shows (state) information of the actor itself. The outputs are position in the experiment's axis system and the GPS coordinates, and the object's absolute velocity and compass heading.
      |
      | For more information, please click Help.
      mask Help: eval('openHelp(462)')
      mask Display: image(imread('GPS.png'))
  SELF_Box_2 : Outport  Tag=outport/SelfPort  OutDataTypeStr=Bus: PRESCAN_SELFSENSORDATA  PortDimensions=1  SampleTime=1/60
  wires:
  Sensor/1 -> SELF_Box_2/1

== system Demo_TA_cs/SELF_Box_3 ==
  Sensor : S-Function  FunctionName=sfun_SelfSensor  Parameters=UniqueID, TimeStep  EnableBusSupport=off  mask(PreScan Source Block: SELF){UniqueID=10, TimeStep=1/60}
      mask prompts: UniqueID "Auto-Assigned: Unique ID"; TimeStep "Auto-Assigned: Upload Period [s]"
      mask help:
      | The SELF port shows (state) information of the actor itself. The outputs are position in the experiment's axis system and the GPS coordinates, and the object's absolute velocity and compass heading.
      |
      | For more information, please click Help.
      mask Help: eval('openHelp(462)')
      mask Display: image(imread('GPS.png'))
  SELF_Box_3 : Outport  Tag=outport/SelfPort  OutDataTypeStr=Bus: PRESCAN_SELFSENSORDATA  PortDimensions=1  SampleTime=1/60
  wires:
  Sensor/1 -> SELF_Box_3/1

== system Demo_TA_cs/SELF_Mazda_RX8_1 ==
  Sensor : S-Function  FunctionName=sfun_SelfSensor  Parameters=UniqueID, TimeStep  EnableBusSupport=off  mask(PreScan Source Block: SELF){UniqueID=6, TimeStep=1/60}
      mask prompts: UniqueID "Auto-Assigned: Unique ID"; TimeStep "Auto-Assigned: Upload Period [s]"
      mask help:
      | The SELF port shows (state) information of the actor itself. The outputs are position in the experiment's axis system and the GPS coordinates, and the object's absolute velocity and compass heading.
      |
      | For more information, please click Help.
      mask Help: eval('openHelp(462)')
      mask Display: image(imread('GPS.png'))
  SELF_Mazda_RX8_1 : Outport  Tag=outport/SelfPort  OutDataTypeStr=Bus: PRESCAN_SELFSENSORDATA  PortDimensions=1  SampleTime=1/60
  wires:
  Sensor/1 -> SELF_Mazda_RX8_1/1

== system Demo_TA_cs/STATE_Box_1_bus ==
  STATE_Box_1_bus : Inport  Tag=inport/StatePort  OutDataTypeStr=Bus: PRESCAN_STATEACTUATORDATA  PortDimensions=1  SampleTime=1/60  BusOutputAsStruct=on
  Actuator : S-Function  FunctionName=sfun_StateActuator  Parameters=UniqueID, TimeStep  EnableBusSupport=off  mask(PreScan Sink Block: State){UniqueID=8, TimeStep=1/60}
      mask prompts: UniqueID "Auto-Assigned: Unique ID"; TimeStep "Auto-Assigned: Upload Period [s]"
      mask help:
      | The Actor State contains a vector signal of size (9x1), containing the following signals:
      |
      | -  Position    	(x,y,z)             	[m]
      | -  Velocity    	(vx,vy,vz)         	[m/s]
      | -  Angles       	(Roll, Pitch, Yaw)	[rad]
      |
      | The Actor state is defined in the global axis system.
      | The state is superponed on the Initial position defined in the GUI.
      |
      | For more information, please click Help.
      mask Help: eval('openHelp(222)')
      mask Display: image(imread('State.png'))
  wires:
  STATE_Box_1_bus/1 -> Actuator/1

== system Demo_TA_cs/STATE_Box_2_bus ==
  STATE_Box_2_bus : Inport  Tag=inport/StatePort  OutDataTypeStr=Bus: PRESCAN_STATEACTUATORDATA  PortDimensions=1  SampleTime=1/60  BusOutputAsStruct=on
  Actuator : S-Function  FunctionName=sfun_StateActuator  Parameters=UniqueID, TimeStep  EnableBusSupport=off  mask(PreScan Sink Block: State){UniqueID=9, TimeStep=1/60}
      mask prompts: UniqueID "Auto-Assigned: Unique ID"; TimeStep "Auto-Assigned: Upload Period [s]"
      mask help:
      | The Actor State contains a vector signal of size (9x1), containing the following signals:
      |
      | -  Position    	(x,y,z)             	[m]
      | -  Velocity    	(vx,vy,vz)         	[m/s]
      | -  Angles       	(Roll, Pitch, Yaw)	[rad]
      |
      | The Actor state is defined in the global axis system.
      | The state is superponed on the Initial position defined in the GUI.
      |
      | For more information, please click Help.
      mask Help: eval('openHelp(222)')
      mask Display: image(imread('State.png'))
  wires:
  STATE_Box_2_bus/1 -> Actuator/1

== system Demo_TA_cs/STATE_Box_3_bus ==
  STATE_Box_3_bus : Inport  Tag=inport/StatePort  OutDataTypeStr=Bus: PRESCAN_STATEACTUATORDATA  PortDimensions=1  SampleTime=1/60  BusOutputAsStruct=on
  Actuator : S-Function  FunctionName=sfun_StateActuator  Parameters=UniqueID, TimeStep  EnableBusSupport=off  mask(PreScan Sink Block: State){UniqueID=10, TimeStep=1/60}
      mask prompts: UniqueID "Auto-Assigned: Unique ID"; TimeStep "Auto-Assigned: Upload Period [s]"
      mask help:
      | The Actor State contains a vector signal of size (9x1), containing the following signals:
      |
      | -  Position    	(x,y,z)             	[m]
      | -  Velocity    	(vx,vy,vz)         	[m/s]
      | -  Angles       	(Roll, Pitch, Yaw)	[rad]
      |
      | The Actor state is defined in the global axis system.
      | The state is superponed on the Initial position defined in the GUI.
      |
      | For more information, please click Help.
      mask Help: eval('openHelp(222)')
      mask Display: image(imread('State.png'))
  wires:
  STATE_Box_3_bus/1 -> Actuator/1

== system Demo_TA_cs/STATE_Mazda_RX8_1_bus ==
  STATE_Mazda_RX8_1_bus : Inport  Tag=inport/StatePort  OutDataTypeStr=Bus: PRESCAN_STATEACTUATORDATA  PortDimensions=1  SampleTime=1/60  BusOutputAsStruct=on
  Actuator : S-Function  FunctionName=sfun_StateActuator  Parameters=UniqueID, TimeStep  EnableBusSupport=off  mask(PreScan Sink Block: State){UniqueID=6, TimeStep=1/60}
      mask prompts: UniqueID "Auto-Assigned: Unique ID"; TimeStep "Auto-Assigned: Upload Period [s]"
      mask help:
      | The Actor State contains a vector signal of size (9x1), containing the following signals:
      |
      | -  Position    	(x,y,z)             	[m]
      | -  Velocity    	(vx,vy,vz)         	[m/s]
      | -  Angles       	(Roll, Pitch, Yaw)	[rad]
      |
      | The Actor state is defined in the global axis system.
      | The state is superponed on the Initial position defined in the GUI.
      |
      | For more information, please click Help.
      mask Help: eval('openHelp(222)')
      mask Display: image(imread('State.png'))
  wires:
  STATE_Mazda_RX8_1_bus/1 -> Actuator/1

== system Demo_TA_cs/ScenarioEngine ==
  Clock : Clock
  sfun_ScenarioEngine : S-Function  FunctionName=sfun_ScenarioEngine  Parameters=TimeStep  EnableBusSupport=off
  wires:
  Clock/1 -> sfun_ScenarioEngine/1

== system Demo_TA_cs/Synchronizer ==
  Bus Selector1 : BusSelector  OutputSignals=FederateStopped
  Stop Simulation : Stop
  sfun_Synchronizer : S-Function  FunctionName=sfun_Synchronizer  Parameters=SampleTime  EnableBusSupport=off  mask(Legacy Function){SFunctionSpec=void prescan_synchronizer_outputFcn(void ** work1, PRESCAN_SYNCHRONIZEDATA y1[1]), SampleTime=TimeStep, ShowSpec=on}
      mask prompts: SampleTime "Sample time (-1 for inherited):"; ShowSpec "Display function specification"
      mask help:
      | This block allows you to call the legacy functions specified by the following Legacy Code Tool definition:
      | def.SFunctionName = 'sfun_Synchronizer';
      | def.OutputFcnSpec = 'void prescan_synchronizer_outputFcn(void ** work1, PRESCAN_SYNCHRONIZEDATA y1[1])';
      | def.StartFcnSpec = 'void prescan_synchronizer_startFcn(void ** work1)';
      | def.TerminateFcnSpec = 'void prescan_synchronizer_terminateFcn(void ** work1)';
      | def.HeaderFiles = {'prescan_synchronizer_data.h'};
      | def.HostLibFiles = {'sensorinterfaced.lib'};
      | def.IncPaths = {'src', 'C:\prescandev\vislibrary\vis\..\pimp\include\sensors\InterfaceRTW'};
      | def.SrcPaths = {'src'};
      | def.LibPaths = {'C:\\prescandev\\vislibrary_build\lib'};
      | def.SampleTime = 'parameterized';
      | def.Options.language = 'C';
      mask Help: <p>This block was generated automatically by the Legacy Code Tool. For detailed help on this tool, call<a href="matlab:legacy_code('help')"> legacy_code('help')</a>.</p>
      mask Callback ShowSpec:
      | if strcmp(get_param(gcbh, 'ShowSpec'), 'on')
      |   set_param(gcbh, 'MaskDisplay', sprintf('fprintf(''%s'');', get_param(gcbh, 'SFunctionSpec')));
      | else
      |   set_param(gcbh, 'MaskDisplay', sprintf('fprintf(''%s'');', get_param(gcbh, 'FunctionName')));
      | end
      mask Display: fprintf('void prescan_synchronizer_outputFcn(void ** work1, PRESCAN_SYNCHRONIZEDATA y1[1])');
  wires:
  Bus Selector1/1 -> Stop Simulation/1  "<FederateStopped>"
  sfun_Synchronizer/1 -> Bus Selector1/1

== system Demo_TA_cs/TIS_1 ==
  Sensor : S-Function  FunctionName=sfun_TIS  Parameters=sensorID, detectableObjects, timestep  EnableBusSupport=off  mask(PreScan Source Block: Technology Independent Sensor (TIS)){sensorID=7, detectableObjects=1, timestep=1/60}
      mask prompts: sensorID "Sensor ID"; detectableObjects "Max detectable objects:"; timestep "MATLAB timestep:"
      mask help:
      | The Technology Independent Sensor (TIS) provides a sensor with all sensor-related influence factors (like noise, drift and accuracy) without being technology specific (like radar and lidar). The TIS detects the closest point on the geometry of an object.
      |
      | For more information, please click Help.
      mask Help: eval('openHelp(449)')
      mask Display: image(imread('TIS.png'))
  TIS_1 : Outport  Tag=outport/TIS  OutDataTypeStr=Bus: PRESCAN_SCANNERSENSOR_MESSAGE  PortDimensions=1  SampleTime=1/60
  wires:
  Sensor/1 -> TIS_1/1

== system Demo_TA_cs/TIS_1_TA ==
  TIS_1_TA : Inport  Tag=inport/TIS_TA  OutDataTypeStr=Bus: PRESCAN_SCANNERSENSOR_TA  PortDimensions=1  SampleTime=1/60  BusOutputAsStruct=on
  Actuator : S-Function  FunctionName=sfun_TIS_TA  Parameters=sensorID, timestep  EnableBusSupport=off  mask(TIS Test Automation){sensorID=7, timestep=1/60}
      mask prompts: sensorID "Sensor ID"; timestep "MATLAB timestep:"
      mask help:
      | The TA Sink block updates the Test Automation variables in the Simulation.
      |
      | Note: All angles are expressed in degrees
      |
      | Remarks:
      | TIS: Drift Type:
      |   0: None
      |   1: Gaussian
      |   2: Unidirectional
      |
      | TIS: Noise Type:
      |   0: Additive
      |   1: Multiplicative
      |
      | AIR: Detection Type:
      |   0: BoundingBox
      |   1: Bounding Box Center
      |   2: CenterOfGravity
      |
      | Antenna Tx: Range
      |   -1: Infinite
      |
      | For more information, please click Help.
      mask Help: eval('openHelp(633)')
      mask Display: image(imread('TA.png'))
  wires:
  TIS_1_TA/1 -> Actuator/1

== system Demo_TA_cs/Box_1/Dynamics_Empty ==
  note: For state mode 'Dynamic' positions
      | are not taken into account, as they
      | are computed by integrating velocity.
      | Click annotation for Help.
  Ground_{1..9} (9 alike) : Ground
  MuxState : Subsystem  Tag=mux/State  mask(Empty Dynamics State Block){positioningmode=on, TimeStep=1/60}
      mask prompts: positioningmode "Positioning Mode"; TimeStep "Auto Assigned: Time Step [s]"
      mask help:
      | Build the state of an actor based on user input.
      | The user can either use positioning mode or dynamics mode.
      | - When using positioning mode the position and orientation of the actor are set directly based on the input. Expected input is relative to the initial position and orientation of the actor. It's also possible to specify the velocity of the actor, though this input isn't used, only passed on.
      | - When using dynamics mode the position input is ignored. Expected input is velocity and orientation. The velocity is relative the current orientation of the actor, while orientation is relative to its initial orientation. The position of the actor is calculated based on the velocity and orientation given.
      settings: DeleteFcn=PreScanBlockDeleteFcn;
  STATE_Box_1 : Subsystem  Tag=mux/StatePort  Priority=0  LoadFcn=load PrescanStateActuatorData  mask(PreScan Sink Block: State){x0=Demo_TA_cs_Box_1_Dynamics_Empty_STATE_Box_1_x0, y0=Demo_TA_cs_Box_1_Dynamics_Empty_STATE_Box_1_y0, z0=Demo_TA_cs_Box_1_Dynamics_Empty_STATE_Box_1_z0, Roll0=Demo_TA_cs_Box_1_Dynamics_Empty_STATE_Box_1_Roll0, Pitch0=Demo_TA_cs_Box_1_Dynamics_Empty_STATE_Box_1_Pitch0, Yaw0=Demo_TA_cs_Box_1_Dynamics_Empty_STATE_Box_1_Yaw0, TimeStep=1/60}
      mask prompts: x0 "Ini x-position VEHICLE wrt GLOBAL axis system [m]"; y0 "Ini y-position VEHICLE wrt GLOBAL axis system [m]"; z0 "Ini z-position VEHICLE wrt GLOBAL axis system [m]"; Roll0 "Ini roll-angle BODY wrt VEHICLE axis system [deg]"; Pitch0 "Ini pitch-angle BODY wrt VEHICLE axis system [deg]"; Yaw0 "Ini yaw-angle VEHICLE wrt GLOBAL axis system [deg]"; TimeStep "Auto-Assigned: Upload Period [s]"
      mask help:
      | The Actor State contains a vector signal of size (9x1), containing the following signals:
      |
      | -  Position                  (x,y,z)                                     [m]
      | -  Velocity                  (vx,vy,vz)                               [m/s]
      | -  Angles                    (Roll, Pitch, Yaw)                   [rad]
      |
      | The Actor state is defined in the global axis system.
      | The state is superponed on the Initial position defined in the GUI.
      |
      | For more information, please click Help.
      settings: DeleteFcn=PreScanBlockDeleteFcn;
      mask Help: eval('openHelp(222)')
      mask Display: image(imread('State.png'))
  State : Outport  Tag=outport/StateOutport  SampleTime=1/60
  wires:
  MuxState/1(state) -> STATE_Box_1/1(State)
  STATE_Box_1/1(StateBus) -> State/1
  Ground_1/1 -> MuxState/1(x [m])
  Ground_2/1 -> MuxState/2(y [m])
  Ground_3/1 -> MuxState/3(z [m])
  Ground_4/1 -> MuxState/4(dx [m/s])
  Ground_5/1 -> MuxState/5(dy [m/s])
  Ground_6/1 -> MuxState/6(dz [m/s])
  Ground_7/1 -> MuxState/7(R [rad])
  Ground_8/1 -> MuxState/8(P [rad])
  Ground_9/1 -> MuxState/9(Y [rad])

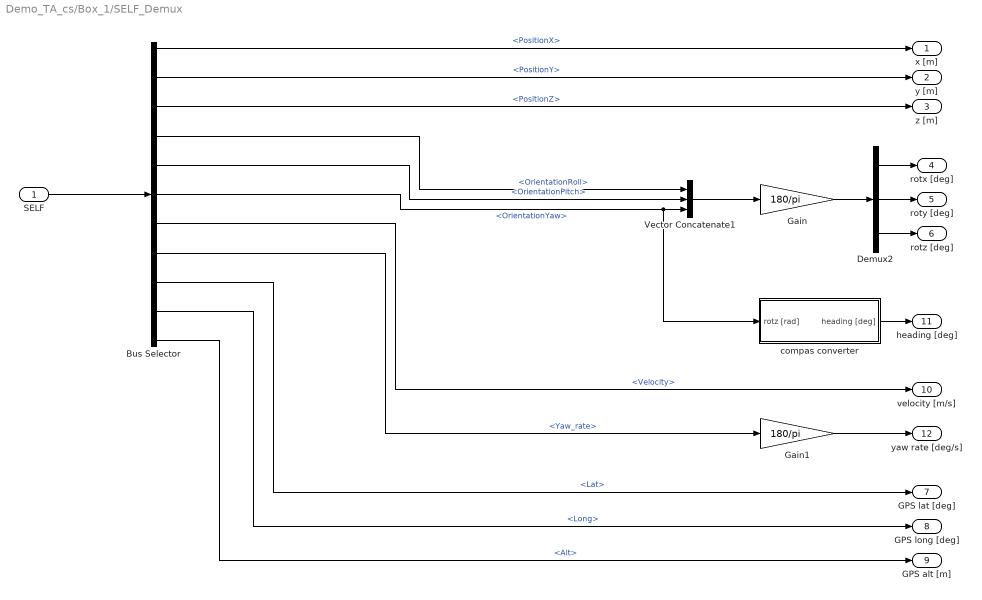
== system Demo_TA_cs/Box_1/SELF_Demux ==
  SELF : Inport  OutDataTypeStr=Bus: PRESCAN_SELFSENSORDATA
  Bus Selector : BusSelector  OutputSignals=PositionX,PositionY,PositionZ,OrientationRoll,OrientationPitch,OrientationYaw,Velocity,Yaw_rate,Lat,Long,Alt
  Demux2 : Demux  Outputs=3
  Gain : Gain  Gain=180/pi
  Gain1 : Gain  Gain=180/pi
  Vector Concatenate1 : Concatenate  NumInputs=3
  compas converter : Subsystem
  x [m] : Outport
  y [m] : Outport  Port=2
  z [m] : Outport  Port=3
  rotx [deg] : Outport  Port=4
  roty [deg] : Outport  Port=5
  rotz [deg] : Outport  Port=6
  GPS lat [deg] : Outport  Port=7
  GPS long [deg] : Outport  Port=8
  GPS alt [m] : Outport  Port=9
  velocity [m/s] : Outport  Port=10
  heading [deg] : Outport  Port=11
  yaw rate [deg/s] : Outport  Port=12
  wires:
  Bus Selector/11 -> GPS alt [m]/1  "<Alt>"
  Bus Selector/10 -> GPS long [deg]/1  "<Long>"
  Bus Selector/9 -> GPS lat [deg]/1  "<Lat>"
  Bus Selector/8 -> Gain1/1  "<Yaw_rate>"
  Bus Selector/7 -> velocity [m/s]/1  "<Velocity>"
  Bus Selector/6 -> compas converter/1(rotz [rad]), Vector Concatenate1/3  "<OrientationYaw>"
  Bus Selector/5 -> Vector Concatenate1/2  "<OrientationPitch>"
  Bus Selector/4 -> Vector Concatenate1/1  "<OrientationRoll>"
  Vector Concatenate1/1 -> Gain/1
  Bus Selector/3 -> z [m]/1  "<PositionZ>"
  Bus Selector/2 -> y [m]/1  "<PositionY>"
  Bus Selector/1 -> x [m]/1  "<PositionX>"
  SELF/1 -> Bus Selector/1
  Gain/1 -> Demux2/1
  Demux2/1 -> rotx [deg]/1
  Demux2/2 -> roty [deg]/1
  Demux2/3 -> rotz [deg]/1
  compas converter/1(heading [deg]) -> heading [deg]/1
  Gain1/1 -> yaw rate [deg/s]/1
